simulink model "pendulum"  (R2020a)
settings: Solver=ode23t  StartTime=0.0  StopTime=4  RelTol=1e-4  AbsTol=1e-6
model workspace (MAT data in the model file):
  L = 1
  g = 9.81
  lambda0 = 0
  m = 1
  omega0 = 0
  theta0 = 1.57079632679
  u0 = 0
  v0 = 0
  x0 = 1
  y0 = 0
settings Model: Creator=The MathWorks, Inc.  LastModifiedBy=The MathWorks, Inc.
settings SolverCC: AutoScaleAbsTol=off  MaxConsecutiveMinStep=3
settings DataIOCC: SaveFormat=Array  TimeSaveName=t  OutputSaveName=y
settings DebuggingCC: AlgebraicLoopMsg=none  ArithmeticOperatorsInVariantConditions=warning
settings SFSimCC: SimUseLocalCustomCode=off  CustomCodeUndefinedFunction=UseInterfaceOnly
settings RTWCC: RTWUseLocalCustomCode=off

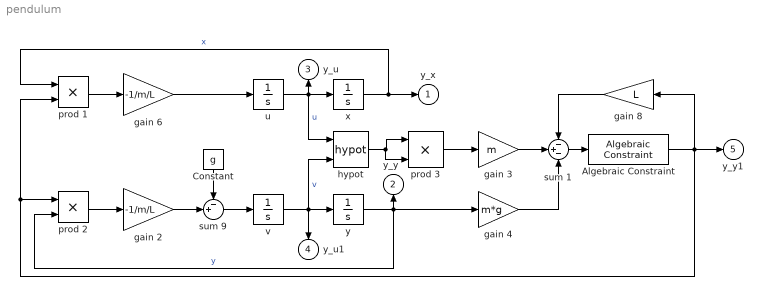
== system pendulum ==
  Algebraic Constraint : AlgebraicConstraint  Solver=Trust region  InitialGuess=-lambda0
  Constant : Constant  Value=g
  gain 2 : Gain  Gain=-1/m/L
  gain 3 : Gain  Gain=m
  gain 4 : Gain  Gain=m*g
  gain 6 : Gain  Gain=-1/m/L
  gain 8 : Gain  Gain=L
  hypot : Math  Operator=hypot  SignedPower=on  SaturateOnIntegerOverflow=on
  prod 1 : Product
  prod 2 : Product
  prod 3 : Product
  sum 1 : Sum  Inputs=-+-
  sum 9 : Sum  Inputs=-+|
  u : Integrator  InitialCondition=u0
  v : Integrator  InitialCondition=v0
  x : Integrator  InitialCondition=x0
  y : Integrator  InitialCondition=y0
  y_x : Outport  VectorParamsAs1DForOutWhenUnconnected=off
  y_y : Outport  Port=2  VectorParamsAs1DForOutWhenUnconnected=off
  y_u : Outport  Port=3  VectorParamsAs1DForOutWhenUnconnected=off
  y_u1 : Outport  Port=4  VectorParamsAs1DForOutWhenUnconnected=off
  y_y1 : Outport  Port=5  VectorParamsAs1DForOutWhenUnconnected=off
  wires:
  sum 1/1 -> Algebraic Constraint/1
  u/1 -> hypot/1, y_u/1, x/1  "u"
  v/1 -> hypot/2, y_u1/1, y/1  "v"
  x/1 -> y_x/1, prod 1/1  "x"
  y/1 -> prod 2/2, gain 4/1, y_y/1  "y"
  gain 6/1 -> u/1
  prod 1/1 -> gain 6/1
  Constant/1 -> sum 9/1
  hypot/1 -> prod 3/2, prod 3/1
  prod 3/1 -> gain 3/1
  gain 3/1 -> sum 1/2
  gain 4/1 -> sum 1/3
  Algebraic Constraint/1 -> y_y1/1, gain 8/1, prod 1/2, prod 2/1
  gain 8/1 -> sum 1/1
  gain 2/1 -> sum 9/2
  prod 2/1 -> gain 2/1
  sum 9/1 -> v/1
